simulink library "arduinoDrivers_lib"  (R2016b)
settings: Solver=ode45  StartTime=0.0  StopTime=10.0  RelTol=1e-3  EnableMultiTasking=on
undefined symbols (not defined in the file or in its folder): tS
libraries: arduinoDrivers_lib x4, arduinolib x2
settings Model: Creator=Raphael  LastModifiedBy=Raphael
settings DataIOCC: LimitDataPoints=on
settings OptimizationCC: LifeSpan=inf
settings DebuggingCC: AllowSymbolicDim=off  SFUnexpectedBacktrackingDiag=warning  SFNoUnconditionalDefaultTransitionDiag=warning  SFExecutionAtInitializationDiag=none
settings GRTTargetCC: TargetLangStandard=C89/C90 (ANSI)  GeneratePreprocessorConditionals=Disable all
settings ConfigComp: CovMetricSettings=dw  CovHtmlReporting=on  CovSaveCumulativeToWorkspaceVar=on  CovSaveSingleToWorkspaceVar=on  CovExternalEMLEnable=off

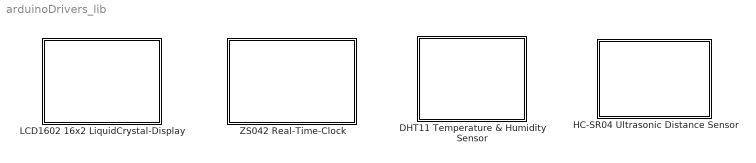
== system arduinoDrivers_lib ==
  DHT11 Temperature & Humidity Sensor : Subsystem
      mask Display: image('.\img\DHT11.jpg');
  HC-SR04 Ultrasonic Distance Sensor : Subsystem
      mask Display: image('.\img\HC-SR04.jpg');
  LCD1602 16x2 LiquidCrystal-Display : Subsystem
      mask Display: image('.\img\LCD1602.jpg');
  ZS042 Real-Time-Clock : Subsystem
      mask Display: image('.\img\ZS-042.png');

== system arduinoDrivers_lib/DHT11 Temperature & Humidity Sensor ==
  DHT11 Temperature & Humidity Sensor : Subsystem  mask(DHT11 Temperature and Humidity Sensor){pin_Mask=1, tS_Mask=1}
      mask prompts: pin_Mask "Pin Number:"; tS_Mask "Sample Time:"
      mask help:
      | Read the temperature in degrees Celcius and the relative humidity from a DHT11 sensor.
      |
      | Output data types: single
      mask TypeOptions tS_Mask: Subsystem/SystemSampleTime

== system arduinoDrivers_lib/HC-SR04 Ultrasonic Distance Sensor ==
  HC-SR04 Ultrasonic Distance Sensor : Subsystem  SystemSampleTime=tS  mask(Get Distance from HC-SR04 Ultrasonic Sensor){trigMask=30, echoMask=31, tsMask=0.5}
      mask prompts: trigMask "Trigger Pin"; echoMask "Echo Pin"; tsMask "Sample Time"
      mask help: When the block is executed, the measured free distance in front of the ultrasonic sensor in centimeters is written to the output port.

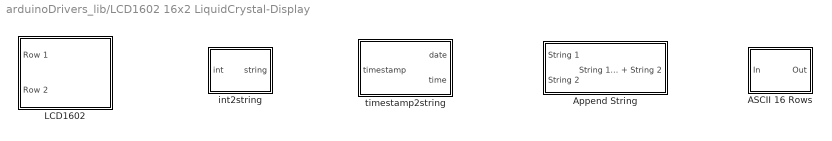
== system arduinoDrivers_lib/LCD1602 16x2 LiquidCrystal-Display ==
  ASCII 16 Rows : Subsystem  mask(Convert to ASCII-Vector with 16 Rows){}
      mask help:
      | The first 16 characters of the input vector are copied into the output vector of data type 'uint8'.
      | If there are less input values the empty fields are filled with 0 = '\0' (String termination).
  Append String : Subsystem  mask(Connect two Texts (ASCII-Vectors)){}
      mask help:
      | The ASCII-vectors at the input ports are connected and present at the output port.
      |
      | Output vector size: 16 characters
  LCD1602 : Subsystem  mask(Driver for 16x2 LiquidCrystal-Display){rsMask=26, enMask=27, d4Mask=22, d5Mask=23, d6Mask=24, d7Mask=25}
      mask prompts: rsMask "RS Pin"; enMask "EN Pin"; d4Mask "D4 Pin"; d5Mask "D5 Pin"; d6Mask "D6 Pin"; d7Mask "D7 Pin"
      mask help:
      | When the block is executed, the ASCII-Vectors at the input ports are printed on the LCD while only the first 16 characters are used.
      |
      | A constant source must be filled like this:
      | 	uint8('TextExample')
      |
      | - Driver works with every Hitachi HD44780-based (or compatible) LC-Display
      | - 16 columns x 2 rows
      | - 4-bit-data mode --> 6 I/O-pins in total (set pin numbers of used pins on Arduino below)
  int2string : Subsystem  mask(Convert Integer to String){}
      mask help: Output vector size: 16 characters
  timestamp2string : Subsystem  mask(Convert Timestamp to Strings){}
      mask help:
      | Input: uint8(sec;min;hour;weekday;day;month;year) as real decimal values.
      | - second:		0 ... 59
      | - minute:		0 ... 59
      | - hour:		0 ... 23
      | - weekday: 	1 ... 7
      | - day:		1 ... 31
      | - month:		1 ... 12
      | - year:		0 ... 99
      |
      | Output:
      | 	DD.MM.YYYY
      | 	HH:MM:SS
      |
      | Output vector sizes: 16 characters

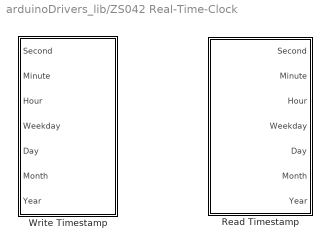
== system arduinoDrivers_lib/ZS042 Real-Time-Clock ==
  Read Timestamp : Subsystem  mask(Read Date and Time from ZS042 Real-Time-Clock){tsMask=1}
      mask prompts: tsMask "Sample Time"
      mask help:
      | This block reads the timestamp from an ZS042 RTC module via I2C-bus.
      |
      | The SCL- and SDA-connections of the module have to be connected to SCL and SDA of the Arduino.
      |
      | Real decimal values are given at the output ports:
      | - second:		0 ... 59
      | - minute:		0 ... 59
      | - hour:		0 ... 23
      | - weekday: 	1 ... 7
      | - day:		1 ... 31
      | - month:		1 ... 12
      | - year:		0 ... 99
  Write Timestamp : Subsystem  mask(Write new Timestamp to ZS042 Real-Time-Clock){}
      mask help:
      | When this block is executed, the values given at the input ports are send to the ZS042 RTC module via I2C-bus.
      |
      | The SCL- and SDA-pins of the module have to be connected to SCL and SDA of the Arduino.
      |
      | Use real decimals as input values:
      | - second:		0 ... 59
      | - minute:		0 ... 59
      | - hour:		0 ... 23
      | - weekday: 	1 ... 7
      | - day:		1 ... 31
      | - month:		1 ... 12
      | - year:		0 ... 99

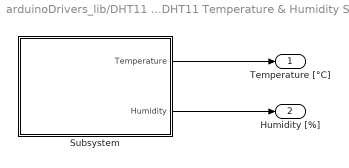
== system arduinoDrivers_lib/DHT11 Temperature & Humidity Sensor/DHT11 Temperature & Humidity Sensor ==
  Subsystem : Subsystem  TreatAsAtomicUnit=on  SystemSampleTime=tS_Mask
  Temperature [°C] : Outport
  Humidity [%] : Outport  Port=2
  wires:
  Subsystem/1(Temperature) -> Temperature [°C]/1
  Subsystem/2(Humidity) -> Humidity [%]/1

== system arduinoDrivers_lib/HC-SR04 Ultrasonic Distance Sensor/HC-SR04 Ultrasonic Distance Sensor ==
  HC-SR04 : Subsystem  TreatAsAtomicUnit=on  SystemSampleTime=tsMask
  Distance [cm] : Outport
  wires:
  HC-SR04/1(Distance) -> Distance [cm]/1

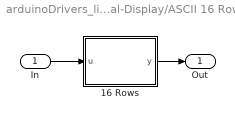
== system arduinoDrivers_lib/LCD1602 16x2 LiquidCrystal-Display/ASCII 16 Rows ==
  In : Inport
  16 Rows : MATLAB Function  TreatAsAtomicUnit=on
  Out : Outport
  wires:
  16 Rows/1(y) -> Out/1
  In/1 -> 16 Rows/1(u)

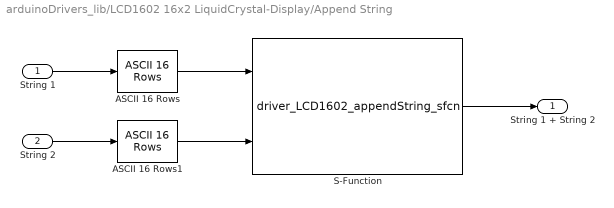
== system arduinoDrivers_lib/LCD1602 16x2 LiquidCrystal-Display/Append String ==
  String 1 : Inport
  String 2 : Inport  Port=2
  ASCII 16 Rows : arduinoDrivers_lib/LCD1602 16x2 LiquidCrystal-Display/ASCII 16 Rows
  ASCII 16 Rows1 : arduinoDrivers_lib/LCD1602 16x2 LiquidCrystal-Display/ASCII 16 Rows
  S-Function : S-Function  FunctionName=driver_LCD1602_appendString_sfcn  SFunctionModules=driver_LCD1602_appendString_sfcn_wrapper  SFunctionDeploymentMode=off  EnableBusSupport=off
  String 1 + String 2 : Outport
  wires:
  S-Function/1 -> String 1 + String 2/1
  String 1/1 -> ASCII 16 Rows/1
  String 2/1 -> ASCII 16 Rows1/1
  ASCII 16 Rows/1 -> S-Function/1
  ASCII 16 Rows1/1 -> S-Function/2

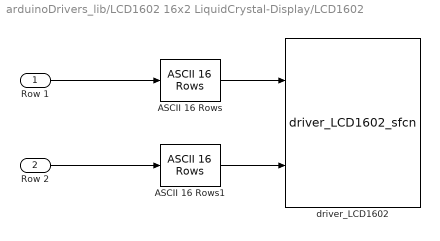
== system arduinoDrivers_lib/LCD1602 16x2 LiquidCrystal-Display/LCD1602 ==
  Row 1 : Inport
  Row 2 : Inport  Port=2
  ASCII 16 Rows : arduinoDrivers_lib/LCD1602 16x2 LiquidCrystal-Display/ASCII 16 Rows
  ASCII 16 Rows1 : arduinoDrivers_lib/LCD1602 16x2 LiquidCrystal-Display/ASCII 16 Rows
  driver_LCD1602 : S-Function  FunctionName=driver_LCD1602_sfcn  Parameters=rsMask,enMask,d4Mask,d5Mask,d6Mask,d7Mask  SFunctionModules=driver_LCD1602_sfcn_wrapper  SFunctionDeploymentMode=off  EnableBusSupport=off
  wires:
  ASCII 16 Rows/1 -> driver_LCD1602/1
  ASCII 16 Rows1/1 -> driver_LCD1602/2
  Row 1/1 -> ASCII 16 Rows/1
  Row 2/1 -> ASCII 16 Rows1/1

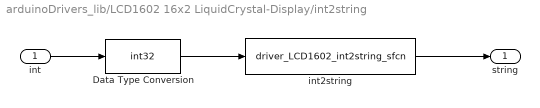
== system arduinoDrivers_lib/LCD1602 16x2 LiquidCrystal-Display/int2string ==
  int : Inport
  Data Type Conversion : DataTypeConversion  OutDataTypeStr=int32
  int2string : S-Function  FunctionName=driver_LCD1602_int2string_sfcn  SFunctionModules=driver_LCD1602_int2string_sfcn_wrapper  SFunctionDeploymentMode=off  EnableBusSupport=off
  string : Outport
  wires:
  int/1 -> Data Type Conversion/1
  Data Type Conversion/1 -> int2string/1
  int2string/1 -> string/1

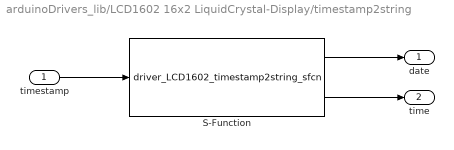
== system arduinoDrivers_lib/LCD1602 16x2 LiquidCrystal-Display/timestamp2string ==
  timestamp : Inport
  S-Function : S-Function  FunctionName=driver_LCD1602_timestamp2string_sfcn  SFunctionModules=driver_LCD1602_timestamp2string_sfcn_wrapper  SFunctionDeploymentMode=off  EnableBusSupport=off
  date : Outport
  time : Outport  Port=2
  wires:
  S-Function/1 -> date/1
  timestamp/1 -> S-Function/1
  S-Function/2 -> time/1

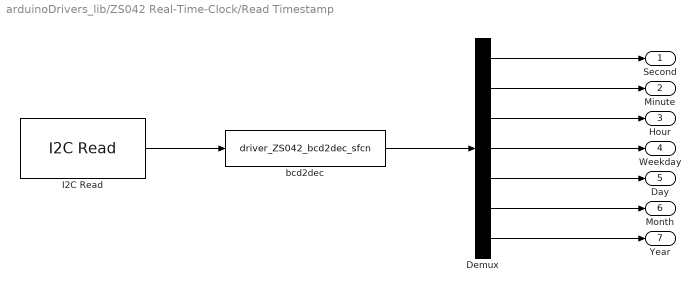
== system arduinoDrivers_lib/ZS042 Real-Time-Clock/Read Timestamp ==
  Demux : Demux  Outputs=7
  I2C Read : arduinolib/I2C Read  SlaveAddress_=hex2dec( '68' )  RegisterAddressEnable=on  RegisterAddress_=hex2dec( '0' )  Datatype=uint8  ByteOrder=Big Endian  Datalength_=7  SampleTime_=tsMask  blockPlatform=arduino
  bcd2dec : S-Function  FunctionName=driver_ZS042_bcd2dec_sfcn  SFunctionModules=driver_ZS042_bcd2dec_sfcn_wrapper  SFunctionDeploymentMode=off  EnableBusSupport=off
  Second : Outport
  Minute : Outport  Port=2
  Hour : Outport  Port=3
  Weekday : Outport  Port=4
  Day : Outport  Port=5
  Month : Outport  Port=6
  Year : Outport  Port=7
  wires:
  I2C Read/1 -> bcd2dec/1
  Demux/5 -> Day/1
  Demux/7 -> Year/1
  Demux/6 -> Month/1
  Demux/1 -> Second/1
  Demux/2 -> Minute/1
  Demux/4 -> Weekday/1
  Demux/3 -> Hour/1
  bcd2dec/1 -> Demux/1

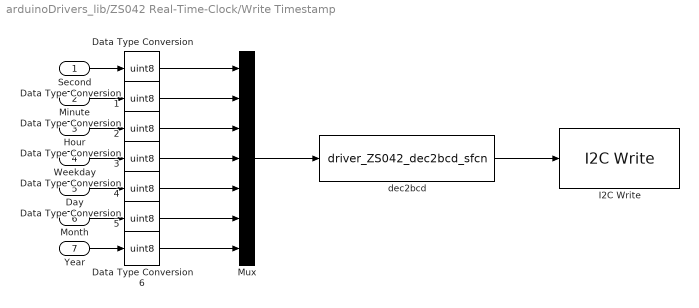
== system arduinoDrivers_lib/ZS042 Real-Time-Clock/Write Timestamp ==
  Second : Inport
  Minute : Inport  Port=2
  Hour : Inport  Port=3
  Weekday : Inport  Port=4
  Day : Inport  Port=5
  Month : Inport  Port=6
  Year : Inport  Port=7
  Data Type Conversion{,1..6} (7 alike) : DataTypeConversion  OutDataTypeStr=uint8
  I2C Write : arduinolib/I2C Write  SlaveAddress_=hex2dec( '68' )  RegisterAddressEnable=on  RegisterAddress_=hex2dec( '0' )  Datatype=uint8  ByteOrder=Big Endian  blockPlatform=arduino
  Mux : Mux  Inputs=7
  dec2bcd : S-Function  FunctionName=driver_ZS042_dec2bcd_sfcn  SFunctionModules=driver_ZS042_dec2bcd_sfcn_wrapper  SFunctionDeploymentMode=off  EnableBusSupport=off
  wires:
  Mux/1 -> dec2bcd/1
  dec2bcd/1 -> I2C Write/1
  Minute/1 -> Data Type Conversion1/1
  Year/1 -> Data Type Conversion6/1
  Second/1 -> Data Type Conversion/1
  Weekday/1 -> Data Type Conversion3/1
  Month/1 -> Data Type Conversion5/1
  Day/1 -> Data Type Conversion4/1
  Hour/1 -> Data Type Conversion2/1
  Data Type Conversion/1 -> Mux/1
  Data Type Conversion1/1 -> Mux/2
  Data Type Conversion2/1 -> Mux/3
  Data Type Conversion3/1 -> Mux/4
  Data Type Conversion4/1 -> Mux/5
  Data Type Conversion5/1 -> Mux/6
  Data Type Conversion6/1 -> Mux/7

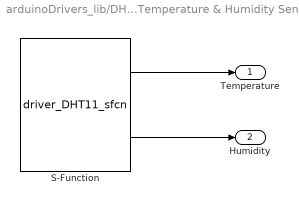
== system arduinoDrivers_lib/DHT11 Temperature & Humidity Sensor/DHT11 Temperature & Humidity Sensor/Subsystem ==
  S-Function : S-Function  FunctionName=driver_DHT11_sfcn  Parameters=uint8(pin_Mask)  SFunctionModules=driver_DHT11_sfcn_wrapper  SFunctionDeploymentMode=off  EnableBusSupport=off
  Temperature : Outport
  Humidity : Outport  Port=2
  wires:
  S-Function/2 -> Humidity/1
  S-Function/1 -> Temperature/1

== system arduinoDrivers_lib/HC-SR04 Ultrasonic Distance Sensor/HC-SR04 Ultrasonic Distance Sensor/HC-SR04 ==
  S-Function : S-Function  FunctionName=driver_HC_SR04_sfcn  Parameters=trigMask,echoMask  SFunctionModules=driver_HC_SR04_sfcn_wrapper  SFunctionDeploymentMode=off  EnableBusSupport=off
  Distance : Outport
  wires:
  S-Function/1 -> Distance/1

== matlab function arduinoDrivers_lib/LCD1602 16x2 LiquidCrystal-Display/ASCII 16 Rows/16 Rows ==
  data: u input; y output size=16
function y = fcn(u)
    y = zeros(16,1,'uint8');
    if(length(u) <= 16)
        y(1:length(u)) = u;
    else
        y(1:16) = u(1:16);
    end
